simulink model "trenl"  (R2021b)
settings: Solver=ode45  StartTime=0.0  StopTime=10.0  RelTol=1e-3  EnableMultiTasking=on
values from neighbouring files (symbols this model uses):
  Am = 1    [treno.m]
  Hz = 0.5    [treno.m]
  NP = 0.2    [treno.m]
  R = b    [treno.m]
  to = round(rand*100)    [treno.m]
  Ts = 0.001    [treno.m]
libraries: commanapbnd3 x2
settings Model: ExtModeTrigDuration=100  Creator=mitrofanova  LastModifiedBy=Вова
settings SolverCC: AlgebraicLoopSolver=TrustRegion
settings DataIOCC: LimitDataPoints=on  SaveFinalState=on  SaveFormat=Array  SignalLoggingSaveFormat=ModelDataLogs  SaveOutput=off  SaveState=on  ReturnWorkspaceOutputs=off  StateSaveName=tmp_raccel_xout  SignalLoggingName=sigsOut
settings OptimizationCC: ExpressionDepthLimit=2147483647  InitFltsAndDblsToZero=on  EfficientMapNaN2IntZero=off  LifeSpan=inf
settings DebuggingCC: SaveWithParameterizedLinksMsg=none  UnderspecifiedInitializationDetection=Classic  MergeDetectMultiDrivingBlocksExec=none  SignalResolutionControl=TryResolveAllWithWarning  MultiTaskDSMMsg=warning  MultiTaskCondExecSysMsg=none  FcnCallInpInsideContextMsg=warning  StateNameClashWarn=warning  SFUnexpectedBacktrackingDiag=warning  SFNoUnconditionalDefaultTransitionDiag=warning  SFExecutionAtInitializationDiag=none  SFMachineParentedDataDiag=warning  ArithmeticOperatorsInVariantConditions=warning
settings HardwareCC: ProdBitPerPointer=32  ProdBitPerSizeT=32  ProdBitPerPtrDiffT=32  ProdLargestAtomicFloat=None  ProdIntDivRoundTo=Undefined  ProdEndianess=Unspecified  ProdWordSize=32  ProdHWDeviceType=32-bit Generic  TargetBitPerPointer=64  TargetBitPerSizeT=64  TargetBitPerPtrDiffT=64  TargetLongLongMode=on  TargetIntDivRoundTo=Zero  TargetEndianess=LittleEndian  TargetWordSize=64  TargetHWDeviceType=MATLAB Host  ProdEqTarget=off
settings ModelReferenceCC: PropagateSignalLabelsOutOfModel=off
settings SFSimCC: SimUseLocalCustomCode=off  CustomCodeUndefinedFunction=UseInterfaceOnly
settings RTWCC: SystemTargetFile=raccel.tlc  TemplateMakefile=raccel_default_tmf  RTWVerbose=off  RTWUseLocalCustomCode=off  RTWUseSimCustomCode=on
settings CodeAppCC: GenerateComments=off  MaxIdLength=128  MangleLength=10  SimulinkBlockComments=off
settings RaccelTargetCC: ParMdlRefBuildCompliant=off  ENABLE_SLEXEC_SSBRIDGE=0  RTWCAPISignals=off  RTWCAPIParams=off  RTWCAPIRootIO=off
settings ConfigComp: CovMetricSettings=dw  CovSaveCumulativeToWorkspaceVar=on  CovSaveSingleToWorkspaceVar=on  CovExternalEMLEnable=off

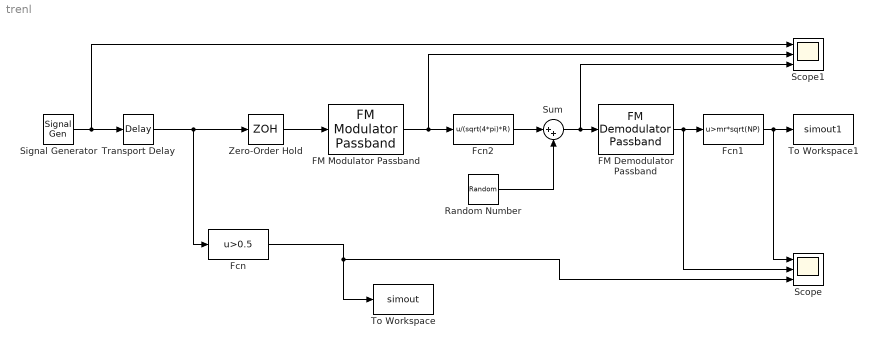
== system trenl ==
  FM Demodulator Passband : commanapbnd3/FM Demodulator Passband  Fc=Fr  Ph=0  Kc=50  Ho=100
      settings: SourceProductBaseCode=CM
  FM Modulator Passband : commanapbnd3/FM Modulator Passband  Fc=Fr  Ph=0  Kc=50
      settings: SourceProductBaseCode=CM
  Fcn : Fcn  Expr=u>0.5  SampleTime=Ts
  Fcn1 : Fcn  Expr=u>mr*sqrt(NP)  SampleTime=Ts
  Fcn2 : Fcn  Expr=u/(sqrt(4*pi)*R)  SampleTime=Ts
  Random Number : RandomNumber  Variance=NP  Seed=to  SampleTime=Ts
  Scope : Scope  NumInputPorts=3
  Scope1 : Scope  NumInputPorts=3
  Signal Generator : SignalGenerator  WaveForm=square  Amplitude=Am  Frequency=Hz
  Sum : Sum  Inputs=|++  SaturateOnIntegerOverflow=on
  To Workspace : ToWorkspace  VariableName=simout  SampleTime=1
  To Workspace1 : ToWorkspace  VariableName=simout1  SampleTime=1
  Transport Delay : TransportDelay  DelayTime=0.1  BufferSize=10240
  Zero-Order Hold : ZeroOrderHold  SampleTime=Ts
  wires:
  Random Number/1 -> Sum/2
  Fcn/1 -> Scope/3, To Workspace/1
  FM Modulator Passband/1 -> Fcn2/1, Scope1/2
  Fcn2/1 -> Sum/1
  Sum/1 -> FM Demodulator Passband/1, Scope1/3
  FM Demodulator Passband/1 -> Fcn1/1, Scope/2
  Fcn1/1 -> Scope/1, To Workspace1/1
  Signal Generator/1 -> Transport Delay/1, Scope1/1
  Transport Delay/1 -> Zero-Order Hold/1, Fcn/1
  Zero-Order Hold/1 -> FM Modulator Passband/1
